simulink model "model_spis"  (R2016b)
settings: Solver=FixedStepDiscrete  StartTime=0.0  StopTime=inf  FixedStep=sampleTime  RelTol=1e-3
PostLoadFcn:
  | parameters_spis;
  | 
  | % set requested state
  | set_param('model_spis/Requested state','Value',num2str(0));
InitFcn:
  | parameters_spis;
  | 
  | % set requested state
  | set_param('model_spis/Requested state','Value',num2str(0));
StartFcn:
  | parameters_spis;
  | 
  | % set requested state
  | set_param('model_spis/Requested state','Value',num2str(0));
undefined symbols (not defined in the file): FM1, FM2, Lb, Lf, Lu, sampleTime
libraries: simulink x29, LibraryFM x14, VariousBlocksLibrary x7, simulink_extras x1
(part 1 of 3)
settings Model: SimulationMode=external  Creator=niekbeckers  LastModifiedBy=Labuser
settings DataIOCC: LimitDataPoints=on  SaveFormat=Array
settings OptimizationCC: BlockReduction=off  BooleanDataType=off  LocalBlockOutputs=off  LifeSpan=inf
settings DebuggingCC: SaveWithParameterizedLinksMsg=none  UnderspecifiedInitializationDetection=Classic  MergeDetectMultiDrivingBlocksExec=none  SignalResolutionControl=TryResolveAllWithWarning  SFUnexpectedBacktrackingDiag=warning  SFNoUnconditionalDefaultTransitionDiag=warning  SFExecutionAtInitializationDiag=none
settings HardwareCC: ProdBitPerPointer=32  ProdBitPerSizeT=32  ProdBitPerPtrDiffT=32  ProdLargestAtomicFloat=None  ProdIntDivRoundTo=Undefined  ProdEndianess=Unspecified  ProdWordSize=32  ProdHWDeviceType=32-bit Generic  TargetBitPerPointer=64  TargetBitPerSizeT=64  TargetBitPerPtrDiffT=64  TargetLongLongMode=on  TargetIntDivRoundTo=Zero  TargetEndianess=LittleEndian  TargetWordSize=64  TargetHWDeviceType=MATLAB Host  ProdEqTarget=off
settings ModelReferenceCC: PropagateSignalLabelsOutOfModel=off
settings RTWCC: SystemTargetFile=TwinCAT.tlc  GenCodeOnly=on  MakeCommand=make_tct  TemplateMakefile=tct_msbuild.tmf  Description=TwinCAT Target  GenerateReport=on  TargetLang=C++
settings STFCustomTargetCC: CompOptLevelCompliant=on  GeneratePreprocessorConditionals=Disable all  MATLABClassNameForMDSCustomization=Simulink.SoftwareTarget.TargetSpecificTriggerConfigurationBase  SystemTargetFile=TwinCAT.tlc
settings ConfigComp: CovMetricSettings=dw  CovHtmlReporting=on  CovSaveCumulativeToWorkspaceVar=on  CovSaveSingleToWorkspaceVar=on  CovExternalEMLEnable=off  CovSFcnEnable=off

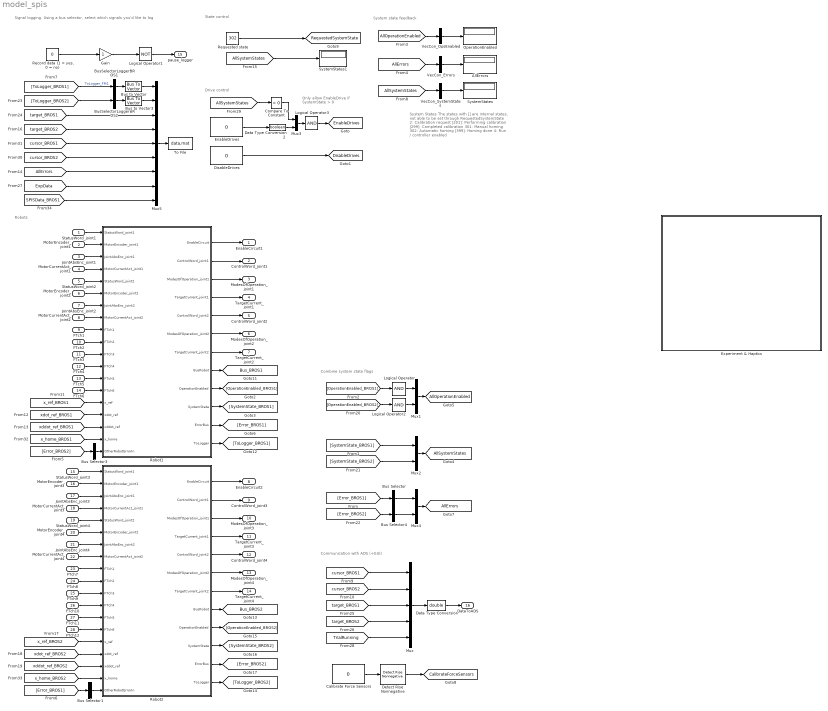
== system model_spis ==
  note: Drive control
  note: System state feedback
  note: Only allow EnableDrive
      | if SystemState > 0
  note: Communication with ADS (+GUI)
  note: Signal logging.
      | Using a bus selector, select which signals you'd like to log
  note: System States
      | The states with [] are internal states, not able to be set through RequestedSystemState
      | 2: Calibration request
      | [201]: Performing calibration
      | [299]: Completed calibration
      | 301: Manual homing
      | 302: Automatic homing
      | [399]: Homing done
      | 4: Run / controller enabled
  note: State control
  note: Combine system state flags
  note: Robots
  StatusWord_joint1 : Inport  OutDataTypeStr=uint16  PortDimensions=1
  MotorEncoder_joint1 : Inport  Port=2  OutDataTypeStr=int32  PortDimensions=1
  JointAbsEnc_joint1 : Inport  Port=3  OutDataTypeStr=int32  PortDimensions=1
  MotorCurrentAct_joint1 : Inport  Port=4  OutDataTypeStr=int16  PortDimensions=1
  StatusWord_joint2 : Inport  Port=5  OutDataTypeStr=uint16  PortDimensions=1
  MotorEncoder_joint2 : Inport  Port=6  OutDataTypeStr=int32  PortDimensions=1
  JointAbsEnc_joint2 : Inport  Port=7  OutDataTypeStr=int32  PortDimensions=1
  MotorCurrentAct_joint2 : Inport  Port=8  OutDataTypeStr=int16  PortDimensions=1
  FTch1 : Inport  Port=9  OutDataTypeStr=single  PortDimensions=1
  FTch2 : Inport  Port=10  OutDataTypeStr=single  PortDimensions=1
  FTch3 : Inport  Port=11  OutDataTypeStr=single  PortDimensions=1
  FTch4 : Inport  Port=12  OutDataTypeStr=single  PortDimensions=1
  FTch5 : Inport  Port=13  OutDataTypeStr=single  PortDimensions=1
  FTch6 : Inport  Port=14  OutDataTypeStr=single  PortDimensions=1
  StatusWord_joint3 : Inport  Port=15  OutDataTypeStr=uint16  PortDimensions=1
  MotorEncoder_joint3 : Inport  Port=16  OutDataTypeStr=int32  PortDimensions=1
  JointAbsEnc_joint3 : Inport  Port=17  OutDataTypeStr=int32  PortDimensions=1
  MotorCurrentAct_joint3 : Inport  Port=18  OutDataTypeStr=int16  PortDimensions=1
  StatusWord_joint4 : Inport  Port=19  OutDataTypeStr=uint16  PortDimensions=1
  MotorEncoder_joint4 : Inport  Port=20  OutDataTypeStr=int32  PortDimensions=1
  JointAbsEnc_joint4 : Inport  Port=21  OutDataTypeStr=int32  PortDimensions=1
  MotorCurrentAct_joint4 : Inport  Port=22  OutDataTypeStr=int16  PortDimensions=1
  FTch7 : Inport  Port=23  OutDataTypeStr=single  PortDimensions=1
  FTch8 : Inport  Port=24  OutDataTypeStr=single  PortDimensions=1
  FTch9 : Inport  Port=25  OutDataTypeStr=single  PortDimensions=1
  FTch10 : Inport  Port=26  OutDataTypeStr=single  PortDimensions=1
  FTch11 : Inport  Port=27  OutDataTypeStr=single  PortDimensions=1
  FTch12 : Inport  Port=28  OutDataTypeStr=single  PortDimensions=1
  AllErrors : Display
  Bus Selector : BusSelector  OutputSignals=ErrorCodeLatched  OutputAsBus=on
  Bus Selector1 : BusSelector  OutputSignals=ErrorCode  OutputAsBus=on
  Bus Selector3 : BusSelector  OutputSignals=ErrorCode  OutputAsBus=on
  Bus Selector4 : BusSelector  OutputSignals=ErrorCodeLatched  OutputAsBus=on
  Bus to Vector : BusToVector
  Bus to Vector3 : BusToVector
  BusSelectorLoggerBROS1 : BusSelector  OutputSignals=SystemState,qJointSpace.q_AbsEnc,qJointSpace.qdot_AbsEnc,qJointSpace.q_IncEnc,qJointSpace.qdot_IncEnc,xOpSpace.x_AbsEnc,xOpSpace.xdot_AbsEnc,Controller_ToLogger.x_ref,Controller_ToLogger.xdot_ref,Controller_ToLogger.xddot_ref,qJointSpace.JointTorque_Nm,BusFTSensor.ForcesOpSpace,BusActuators.BusActuator1.JointVelocity_LPF_rads,BusActuators.BusActuator2.JointVelocity_LPF_rads  OutputAsBus=on
  BusSelectorLoggerBROS2 : BusSelector  OutputSignals=SystemState,qJointSpace.q_AbsEnc,qJointSpace.qdot_AbsEnc,qJointSpace.q_IncEnc,qJointSpace.qdot_IncEnc,xOpSpace.x_AbsEnc,xOpSpace.xdot_AbsEnc,Controller_ToLogger.x_ref,Controller_ToLogger.xdot_ref,Controller_ToLogger.xddot_ref,qJointSpace.JointTorque_Nm,BusFTSensor.ForcesOpSpace,BusActuators.BusActuator1.JointVelocity_LPF_rads,BusActuators.BusActuator2.JointVelocity_LPF_rads  OutputAsBus=on
  Calibrate Force Sensors : Constant  Value=0
      settings: OpenFcn=set_param(gcb,'Value','1');tname = ['toggletimer_' gcb];delete(timerfind('name',tname));t = timer('timerfcn', ['set_param(''',gcb,''',''Value'',''0'')'],'executionmode','singleshot','startdelay',1,'name',tname);start(t);
      mask Display: fprintf('PushToTrigger\n%s',get_param(gcb,'value'))
  Compare To Constant : simulink/Logic and Bit Operations/Compare To Constant  relop=>  const=0  OutDataTypeStr=boolean
  Data Type Conversion : DataTypeConversion  OutDataTypeStr=double
  Data Type Conversion2 : DataTypeConversion  OutDataTypeStr=boolean
  Detect Rise Nonnegative : simulink/Logic and Bit Operations/Detect Rise Nonnegative  vinit=0  OutDataTypeStr=boolean
  DisableDrives : Constant  Value=0
      settings: OpenFcn=set_param(gcb,'Value','1');tname = ['toggletimer_' gcb];delete(timerfind('name',tname));t = timer('timerfcn', ['set_param(''',gcb,''',''Value'',''0'')'],'executionmode','singleshot','startdelay',1,'name',tname);start(t);
      mask Display: fprintf('PushToTrigger\n%s',get_param(gcb,'value'))
  EnableDrives : Constant  Value=0
      settings: OpenFcn=set_param(gcb,'Value','1');tname = ['toggletimer_' gcb];delete(timerfind('name',tname));t = timer('timerfcn', ['set_param(''',gcb,''',''Value'',''0'')'],'executionmode','singleshot','startdelay',1,'name',tname);start(t);
      mask Display: fprintf('PushToTrigger\n%s',get_param(gcb,'value'))
  Experiment & Haptics : Subsystem
  Gain : Gain
  Logical Operator : Logic  Inputs=1  AllPortsSameDT=off  OutDataTypeStr=boolean
  Logical Operator1 : Logic  Operator=NOT  Inputs=1  AllPortsSameDT=off  OutDataTypeStr=boolean
  Logical Operator2 : Logic  Inputs=1  AllPortsSameDT=off  OutDataTypeStr=boolean
  Logical Operator3 : Logic  Inputs=1  AllPortsSameDT=off  OutDataTypeStr=boolean
  Mux : Mux  Inputs=5
  Mux{1..4} (4 alike) : Mux  Inputs=2
  Mux5 : Mux  Inputs=9
  OperationEnabled : Display
  "Record data (1 = yes, 0 = no)" : Constant  Value=0
  Requested state : Constant  Value=302
  Robot1 : Subsystem  mask{RobotStruct=FM1}
      mask prompts: RobotStruct "Robot struct (data)"
  Robot2 : Subsystem  mask{RobotStruct=FM2}
      mask prompts: RobotStruct "Robot struct (data)"
  SystemStates : Display
  SystemStates1 : Display
  To File : ToFile  Filename=data.mat  MatrixName=data
  VecCon_Errors : Concatenate  NumInputs=1
  VecCon_OpsEnabled : Concatenate  NumInputs=1
  VecCon_SystemStates : Concatenate  NumInputs=1
  EnableCircuit1 : Outport  OutDataTypeStr=boolean  PortDimensions=1
  ControlWord_joint1 : Outport  Port=2  OutDataTypeStr=uint16  PortDimensions=1
  ModesOfOperation_joint1 : Outport  Port=3  OutDataTypeStr=int8  PortDimensions=1
  TargetCurrent_joint1 : Outport  Port=4  OutDataTypeStr=int16  PortDimensions=1
  ControlWord_joint2 : Outport  Port=5  OutDataTypeStr=uint16  PortDimensions=1
  ModesOfOperation_joint2 : Outport  Port=6  OutDataTypeStr=int8  PortDimensions=1
  TargetCurrent_joint2 : Outport  Port=7  OutDataTypeStr=int16  PortDimensions=1
  EnableCircuit2 : Outport  Port=8  OutDataTypeStr=boolean  PortDimensions=1
  ControlWord_joint3 : Outport  Port=9  OutDataTypeStr=uint16  PortDimensions=1
  ModesOfOperation_joint3 : Outport  Port=10  OutDataTypeStr=int8  PortDimensions=1
  TargetCurrent_joint3 : Outport  Port=11  OutDataTypeStr=int16  PortDimensions=1
  ControlWord_joint4 : Outport  Port=12  OutDataTypeStr=uint16  PortDimensions=1
  ModesOfOperation_joint4 : Outport  Port=13  OutDataTypeStr=int8  PortDimensions=1
  TargetCurrent_joint4 : Outport  Port=14  OutDataTypeStr=int16  PortDimensions=1
  pause_logger : Outport  Port=15  OutDataTypeStr=boolean  PortDimensions=1
  DataToADS : Outport  Port=16  OutDataTypeStr=double
  tag scope: AllErrors=global, AllOperationEnabled=global, AllSystemStates=global, Bus_BROS1=global, Bus_BROS2=global, CalibrateForceSensors=global, DisableDrives=global, EnableDrives=global, RequestedSystemState=global
  wires:
  DisableDrives/1 -> [DisableDrives]
  Robot1/9(OperationEnabled) -> [OperationEnabled_BROS1]
  [AllOperationEnabled] -> VecCon_OpsEnabled/1
  Robot1/10(SystemState) -> [SystemState_BROS1]
  [SystemState_BROS1] -> Mux2/1
  Mux2/1 -> [AllSystemStates]
  Mux1/1 -> [AllOperationEnabled]
  [OperationEnabled_BROS1] -> Logical Operator/1
  Robot1/11(ErrorBus) -> [Error_BROS1]
  [Error_BROS1] -> Bus Selector/1
  [AllErrors] -> VecCon_Errors/1
  [x_ref_BROS1] -> Robot1/15(x_ref)
  [xdot_ref_BROS1] -> Robot1/16(xdot_ref)
  [xddot_ref_BROS1] -> Robot1/17(xddot_ref)
  Requested state/1 -> [RequestedSystemState]
  Robot1/8(BusRobot) -> [Bus_BROS1]
  StatusWord_joint1/1 -> Robot1/1(StatusWord_joint1)
  MotorEncoder_joint1/1 -> Robot1/2(MotorEncoder_joint1)
  JointAbsEnc_joint1/1 -> Robot1/3(JointAbsEnc_joint1)
  MotorCurrentAct_joint1/1 -> Robot1/4(MotorCurrentAct_joint1)
  StatusWord_joint2/1 -> Robot1/5(StatusWord_joint2)
  MotorEncoder_joint2/1 -> Robot1/6(MotorEncoder_joint2)
  JointAbsEnc_joint2/1 -> Robot1/7(JointAbsEnc_joint2)
  MotorCurrentAct_joint2/1 -> Robot1/8(MotorCurrentAct_joint2)
  FTch1/1 -> Robot1/9(FTch1)
  FTch2/1 -> Robot1/10(FTch2)
  FTch3/1 -> Robot1/11(FTch3)
  FTch4/1 -> Robot1/12(FTch4)
  FTch5/1 -> Robot1/13(FTch5)
  FTch6/1 -> Robot1/14(FTch6)
  Robot1/2(ControlWord_joint1) -> ControlWord_joint1/1
  Robot1/3(ModesOfOperation_joint1) -> ModesOfOperation_joint1/1
  Robot1/4(TargetCurrent_joint1) -> TargetCurrent_joint1/1
  Robot1/7(TargetCurrent_joint2) -> TargetCurrent_joint2/1
  Robot1/6(ModesOfOperation_joint2) -> ModesOfOperation_joint2/1
  Robot1/5(ControlWord_joint2) -> ControlWord_joint2/1
  Robot1/12(ToLogger) -> [ToLogger_BROS1]
  [ToLogger_BROS1] -> BusSelectorLoggerBROS1/1  "ToLogger_FM1"
  Logical Operator/1 -> Mux1/1
  [AllSystemStates] -> SystemStates1/1
  Logical Operator1/1 -> pause_logger/1
  BusSelectorLoggerBROS1/1 -> Bus to Vector/1
  Robot2/9(OperationEnabled) -> [OperationEnabled_BROS2]
  Robot2/10(SystemState) -> [SystemState_BROS2]
  Robot2/11(ErrorBus) -> [Error_BROS2]
  [x_ref_BROS2] -> Robot2/15(x_ref)
  [xdot_ref_BROS2] -> Robot2/16(xdot_ref)
  [xddot_ref_BROS2] -> Robot2/17(xddot_ref)
  Robot2/8(BusRobot) -> [Bus_BROS2]
  StatusWord_joint3/1 -> Robot2/1(StatusWord_joint1)
  MotorEncoder_joint3/1 -> Robot2/2(MotorEncoder_joint1)
  JointAbsEnc_joint3/1 -> Robot2/3(JointAbsEnc_joint1)
  MotorCurrentAct_joint3/1 -> Robot2/4(MotorCurrentAct_joint1)
  StatusWord_joint4/1 -> Robot2/5(StatusWord_joint2)
  MotorEncoder_joint4/1 -> Robot2/6(MotorEncoder_joint2)
  MotorCurrentAct_joint4/1 -> Robot2/8(MotorCurrentAct_joint2)
  FTch7/1 -> Robot2/9(FTch1)
  FTch8/1 -> Robot2/10(FTch2)
  FTch9/1 -> Robot2/11(FTch3)
  FTch10/1 -> Robot2/12(FTch4)
  FTch12/1 -> Robot2/14(FTch6)
  Robot2/1(EnableCircuit) -> EnableCircuit2/1
  Robot2/2(ControlWord_joint1) -> ControlWord_joint3/1
  Robot2/3(ModesOfOperation_joint1) -> ModesOfOperation_joint3/1
  Robot2/7(TargetCurrent_joint2) -> TargetCurrent_joint4/1
  Robot2/6(ModesOfOperation_joint2) -> ModesOfOperation_joint4/1
  Robot2/5(ControlWord_joint2) -> ControlWord_joint4/1
  Robot2/12(ToLogger) -> [ToLogger_BROS2]
  [OperationEnabled_BROS2] -> Logical Operator2/1
  Logical Operator2/1 -> Mux1/2
  [SystemState_BROS2] -> Mux2/2
  Mux4/1 -> [AllErrors]
  Bus Selector/1 -> Mux4/1
  [Error_BROS2] -> Bus Selector4/1
  Bus Selector4/1 -> Mux4/2
  [ToLogger_BROS2] -> BusSelectorLoggerBROS2/1
  BusSelectorLoggerBROS2/1 -> Bus to Vector3/1
  Bus to Vector3/1 -> Mux5/2
  Bus to Vector/1 -> Mux5/1
  Mux5/1 -> To File/1
  Robot1/1(EnableCircuit) -> EnableCircuit1/1
  Robot2/4(TargetCurrent_joint1) -> TargetCurrent_joint3/1
  JointAbsEnc_joint4/1 -> Robot2/7(JointAbsEnc_joint2)
  FTch11/1 -> Robot2/13(FTch5)
  [Error_BROS2] -> Bus Selector3/1
  [Error_BROS1] -> Bus Selector1/1
  Bus Selector1/1 -> Robot2/19(OtherRobotErrorIn)
  Bus Selector3/1 -> Robot1/19(OtherRobotErrorIn)
  VecCon_Errors/1 -> AllErrors/1
  [AllSystemStates] -> VecCon_SystemStates/1
  VecCon_SystemStates/1 -> SystemStates/1
  VecCon_OpsEnabled/1 -> OperationEnabled/1
  Mux/1 -> Data Type Conversion/1
  Data Type Conversion/1 -> DataToADS/1
  [cursor_BROS1] -> Mux/1
  [cursor_BROS2] -> Mux/2
  [target_BROS1] -> Mux/3
  [target_BROS2] -> Mux/4
  [TrialRunning] -> Mux/5
  Calibrate Force Sensors/1 -> Detect Rise Nonnegative/1
  Detect Rise Nonnegative/1 -> [CalibrateForceSensors]
  [target_BROS1] -> Mux5/3
  [AllErrors] -> Mux5/7
  [ExpData] -> Mux5/8
  [target_BROS2] -> Mux5/4
  [AllSystemStates] -> Compare To Constant/1
  Logical Operator3/1 -> [EnableDrives]
  EnableDrives/1 -> Data Type Conversion2/1
  Compare To Constant/1 -> Mux3/1
  Mux3/1 -> Logical Operator3/1
  Data Type Conversion2/1 -> Mux3/2
  [cursor_BROS2] -> Mux5/6
  [cursor_BROS1] -> Mux5/5
  [x_home_BROS1] -> Robot1/18(x_home)
  [x_home_BROS2] -> Robot2/18(x_home)
  "Record data (1 = yes, 0 = no)"/1 -> Gain/1
  Gain/1 -> Logical Operator1/1
  [SPISData_BROS1] -> Mux5/9

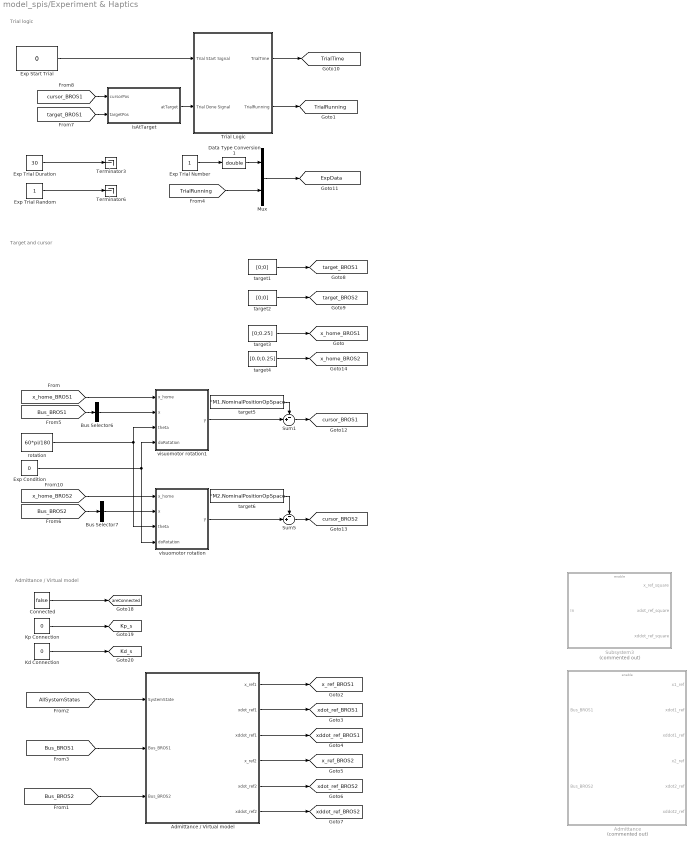
== system model_spis/Experiment & Haptics ==
  note: Target and cursor
  note: Trial logic
  note: Admittance / Virtual model
  Admittance : Subsystem  Commented=on
  Admittance / Virtual model : Subsystem
  Bus Selector6 : BusSelector  OutputSignals=xOpSpace.x  OutputAsBus=on
  Bus Selector7 : BusSelector  OutputSignals=xOpSpace.x  OutputAsBus=on
  Connected : Constant  Value=false  OutDataTypeStr=boolean
  Data Type Conversion1 : DataTypeConversion  OutDataTypeStr=double
  Exp Condition : Constant  Value=0  OutDataTypeStr=int32
  Exp Start Trial : Constant  Value=0
      settings: OpenFcn=set_param(gcb,'Value','1');tname = ['toggletimer_' gcb];delete(timerfind('name',tname));t = timer('timerfcn', ['set_param(''',gcb,''',''Value'',''0'')'],'executionmode','singleshot','startdelay',1,'name',tname);start(t);
      mask Display: fprintf('PushToTrigger\n%s',get_param(gcb,'value'))
  Exp Trial Duration : Constant  Value=30  OutDataTypeStr=double
  Exp Trial Number : Constant  OutDataTypeStr=int32
  Exp Trial Random : Constant  OutDataTypeStr=int32
  Kd Connection : Constant  Value=0  OutDataTypeStr=double
  Kp Connection : Constant  Value=0  OutDataTypeStr=double
  Mux : Mux  Inputs=2
  Subsystem3 : Subsystem  Commented=on
  Sum1 : Sum  Inputs=-+|
  Sum5 : Sum  Inputs=-+|
  Terminator3 : Terminator
  Terminator6 : Terminator
  Trial Logic : Subsystem
  isAtTarget : MATLAB Function  TreatAsAtomicUnit=on
  rotation : Constant  Value=60*pi/180  OutDataTypeStr=double
  target1 : Constant  Value=[0;0]
  target2 : Constant  Value=[0;0]
  target3 : Constant  Value=[0;0.25]
  target4 : Constant  Value=[0.0;0.25]
  target5 : Constant  Value=FM1.NominalPositionOpSpace
  target6 : Constant  Value=FM2.NominalPositionOpSpace
  visuomotor rotation : MATLAB Function  TreatAsAtomicUnit=on
  visuomotor rotation1 : MATLAB Function  TreatAsAtomicUnit=on
  tag scope: ExpData=global, Kd_s=global, Kp_s=global, TrialRunning=global, TrialTime=global, areConnected=global, cursor_BROS1=global, cursor_BROS2=global, target_BROS1=global, target_BROS2=global, x_home_BROS1=global, x_home_BROS2=global, x_ref_BROS1=global, x_ref_BROS2=global, xddot_ref_BROS1=global, xddot_ref_BROS2=global, xdot_ref_BROS1=global, xdot_ref_BROS2=global
  wires:
  target2/1 -> [target_BROS2]
  Kp Connection/1 -> [Kp_s]
  Mux/1 -> [ExpData]
  Exp Trial Number/1 -> Data Type Conversion1/1
  [TrialRunning] -> Mux/2
  Connected/1 -> [areConnected]
  Exp Trial Random/1 -> Terminator6/1
  Data Type Conversion1/1 -> Mux/1
  Kd Connection/1 -> [Kd_s]
  [Bus_BROS1] -> Admittance / Virtual model/2(Bus_BROS1)
  [AllSystemStates] -> Admittance / Virtual model/1(SystemState)
  [Bus_BROS1] -> Bus Selector6/1
  [Bus_BROS2] -> Bus Selector7/1
  Exp Condition/1 -> visuomotor rotation1/4(doRotation), visuomotor rotation/4(doRotation)
  rotation/1 -> visuomotor rotation1/3(theta), visuomotor rotation/3(theta)
  Exp Trial Duration/1 -> Terminator3/1
  Bus Selector6/1 -> visuomotor rotation1/2(x)
  Bus Selector7/1 -> visuomotor rotation/2(x)
  [x_home_BROS1] -> visuomotor rotation1/1(x_home)
  target1/1 -> [target_BROS1]
  target3/1 -> [x_home_BROS1]
  target4/1 -> [x_home_BROS2]
  Exp Start Trial/1 -> Trial Logic/1(Trial Start Signal)
  Trial Logic/1(TrialTime) -> [TrialTime]
  Trial Logic/2(TrialRunning) -> [TrialRunning]
  [cursor_BROS1] -> isAtTarget/1(cursorPos)
  [target_BROS1] -> isAtTarget/2(targetPos)
  isAtTarget/1(atTarget) -> Trial Logic/2(Trial Done Signal)
  [Bus_BROS2] -> Admittance / Virtual model/3(Bus_BROS2)
  Admittance / Virtual model/1(x_ref1) -> [x_ref_BROS1]
  Admittance / Virtual model/2(xdot_ref1) -> [xdot_ref_BROS1]
  Admittance / Virtual model/3(xddot_ref1) -> [xddot_ref_BROS1]
  Admittance / Virtual model/4(x_ref2) -> [x_ref_BROS2]
  Admittance / Virtual model/5(xdot_ref2) -> [xdot_ref_BROS2]
  Admittance / Virtual model/6(xddot_ref2) -> [xddot_ref_BROS2]
  Sum1/1 -> [cursor_BROS1]
  visuomotor rotation/1(y) -> Sum5/2
  target6/1 -> Sum5/1
  Sum5/1 -> [cursor_BROS2]
  [x_home_BROS2] -> visuomotor rotation/1(x_home)
  visuomotor rotation1/1(y) -> Sum1/2
  target5/1 -> Sum1/1

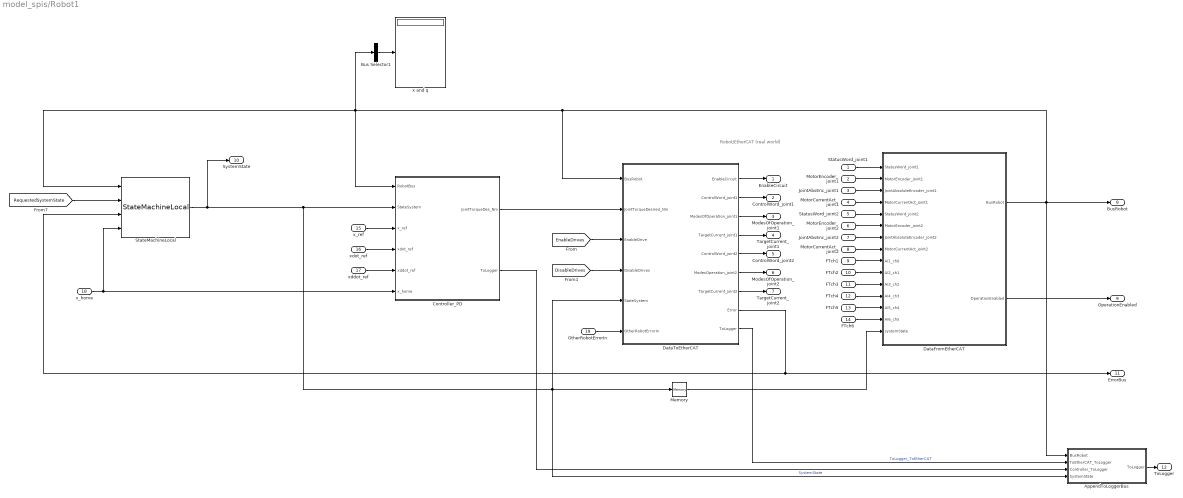
== system model_spis/Robot1 ==
  note: Robot/EtherCAT (real world)
  StatusWord_joint1 : Inport
  MotorEncoder_joint1 : Inport  Port=2
  JointAbsEnc_joint1 : Inport  Port=3
  MotorCurrentAct_joint1 : Inport  Port=4
  StatusWord_joint2 : Inport  Port=5
  MotorEncoder_joint2 : Inport  Port=6
  JointAbsEnc_joint2 : Inport  Port=7
  MotorCurrentAct_joint2 : Inport  Port=8
  FTch1 : Inport  Port=9
  FTch2 : Inport  Port=10
  FTch3 : Inport  Port=11
  FTch4 : Inport  Port=12
  FTch5 : Inport  Port=13
  FTch6 : Inport  Port=14
  x_ref : Inport  Port=15
  xdot_ref : Inport  Port=16
  xddot_ref : Inport  Port=17
  x_home : Inport  Port=18
  OtherRobotErrorIn : Inport  Port=19
  AppendToLoggerBus : Subsystem
  Bus Selector1 : BusSelector  OutputSignals=qJointSpace.q_AbsEnc,qJointSpace.qdot_AbsEnc,xOpSpace.x,BusActuators.BusActuator1.JointPosition_AbsEnc_rad,BusActuators.BusActuator2.JointPosition_AbsEnc_rad  OutputAsBus=on
  Controller_PD : Subsystem
  DataFromEtherCAT : Subsystem
  DataToEtherCAT : Subsystem
  Memory : Memory
  StateMachineLocal : LibraryFM/StateMachineLocal
  x and q : Display
  EnableCircuit : Outport
  ControlWord_joint1 : Outport  Port=2
  ModesOfOperation_joint1 : Outport  Port=3
  TargetCurrent_joint1 : Outport  Port=4
  ControlWord_joint2 : Outport  Port=5
  ModesOfOperation_joint2 : Outport  Port=6
  TargetCurrent_joint2 : Outport  Port=7
  BusRobot : Outport  Port=8
  OperationEnabled : Outport  Port=9
  SystemState : Outport  Port=10
  ErrorBus : Outport  Port=11
  ToLogger : Outport  Port=12
  wires:
  xddot_ref/1 -> Controller_PD/5(xddot_ref)
  xdot_ref/1 -> Controller_PD/4(xdot_ref)
  x_ref/1 -> Controller_PD/3(x_ref)
  DataToEtherCAT/7(TargetCurrent_joint2) -> TargetCurrent_joint2/1
  FTch2/1 -> DataFromEtherCAT/10(AI2_ch1)
  MotorCurrentAct_joint1/1 -> DataFromEtherCAT/4(MotorCurrentAct_joint1)
  MotorEncoder_joint2/1 -> DataFromEtherCAT/6(MotorEncoder_joint2)
  JointAbsEnc_joint1/1 -> DataFromEtherCAT/3(JointAbsoluteEncoder_joint1)
  DataToEtherCAT/3(ModesOfOperation_joint1) -> ModesOfOperation_joint1/1
  DataToEtherCAT/1(EnableCircuit) -> EnableCircuit/1
  FTch1/1 -> DataFromEtherCAT/9(AI1_ch0)
  StateMachineLocal/1 -> Controller_PD/2(StateSystem), DataToEtherCAT/5(StateSystem), Memory/1, AppendToLoggerBus/4(SystemState), SystemState/1  "SystemState"
  DataToEtherCAT/2(ControlWord_joint1) -> ControlWord_joint1/1
  DataToEtherCAT/8(Error) -> StateMachineLocal/3, ErrorBus/1
  DataFromEtherCAT/1(BusRobot) -> AppendToLoggerBus/1(BusRobot), Controller_PD/1(RobotBus), Bus Selector1/1, StateMachineLocal/1, DataToEtherCAT/1(BusRobot), BusRobot/1
  [RequestedSystemState] -> StateMachineLocal/2
  Controller_PD/1(JointTorqueDes_Nm) -> DataToEtherCAT/2(JointTorqueDesired_Nm)
  [DisableDrives] -> DataToEtherCAT/4(DisableDrives)
  [EnableDrives] -> DataToEtherCAT/3(EnableDrive)
  MotorCurrentAct_joint2/1 -> DataFromEtherCAT/8(MotorCurrentAct_joint2)
  DataToEtherCAT/4(TargetCurrent_joint1) -> TargetCurrent_joint1/1
  FTch5/1 -> DataFromEtherCAT/13(AI5_ch4)
  JointAbsEnc_joint2/1 -> DataFromEtherCAT/7("JointAbsoluteEncoder_joint2 ")
  MotorEncoder_joint1/1 -> DataFromEtherCAT/2(MotorEncoder_joint1)
  DataToEtherCAT/5(ControlWord_joint2) -> ControlWord_joint2/1
  DataToEtherCAT/6(ModesOperation_joint2) -> ModesOfOperation_joint2/1
  StatusWord_joint1/1 -> DataFromEtherCAT/1(StatusWord_joint1)
  StatusWord_joint2/1 -> DataFromEtherCAT/5(StatusWord_joint2)
  FTch6/1 -> DataFromEtherCAT/14(AI6_ch5)
  FTch4/1 -> DataFromEtherCAT/12(AI4_ch3)
  FTch3/1 -> DataFromEtherCAT/11(AI3_ch2)
  DataFromEtherCAT/2(OperationEnabled) -> OperationEnabled/1
  Bus Selector1/1 -> x and q/1
  Controller_PD/2(ToLogger) -> AppendToLoggerBus/3(Controller_ToLogger)
  DataToEtherCAT/9(ToLogger) -> AppendToLoggerBus/2(ToEtherCAT_ToLogger)  "ToLogger_ToEtherCAT"
  AppendToLoggerBus/1(ToLogger) -> ToLogger/1
  Memory/1 -> DataFromEtherCAT/15(systemState)
  OtherRobotErrorIn/1 -> DataToEtherCAT/6(OtherRobotErrorIn)
  x_home/1 -> StateMachineLocal/4, Controller_PD/6(x_home)

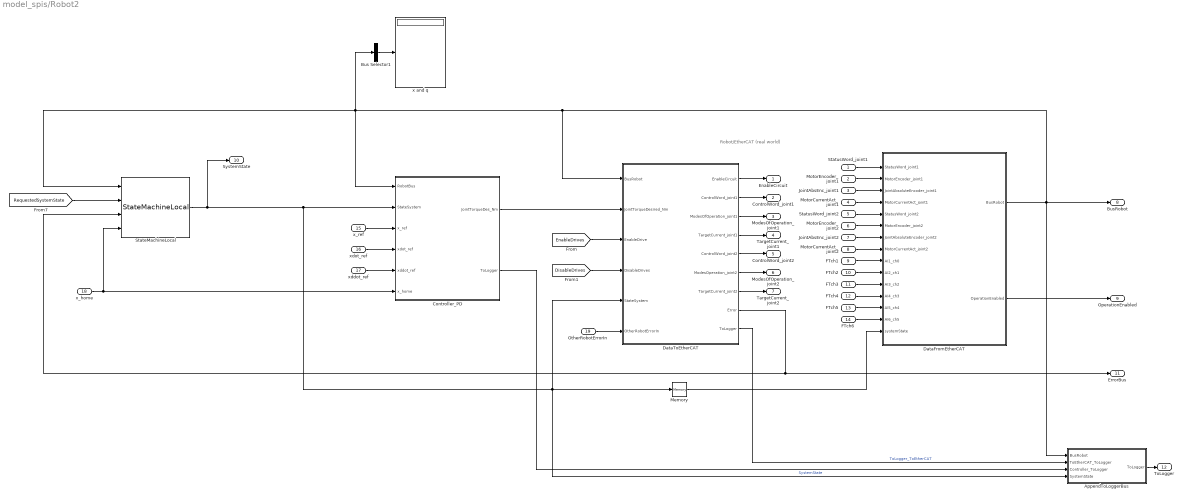
== system model_spis/Robot2 ==
  note: Robot/EtherCAT (real world)
  StatusWord_joint1 : Inport
  MotorEncoder_joint1 : Inport  Port=2
  JointAbsEnc_joint1 : Inport  Port=3
  MotorCurrentAct_joint1 : Inport  Port=4
  StatusWord_joint2 : Inport  Port=5
  MotorEncoder_joint2 : Inport  Port=6
  JointAbsEnc_joint2 : Inport  Port=7
  MotorCurrentAct_joint2 : Inport  Port=8
  FTch1 : Inport  Port=9
  FTch2 : Inport  Port=10
  FTch3 : Inport  Port=11
  FTch4 : Inport  Port=12
  FTch5 : Inport  Port=13
  FTch6 : Inport  Port=14
  x_ref : Inport  Port=15
  xdot_ref : Inport  Port=16
  xddot_ref : Inport  Port=17
  x_home : Inport  Port=18
  OtherRobotErrorIn : Inport  Port=19
  AppendToLoggerBus : Subsystem
  Bus Selector1 : BusSelector  OutputSignals=qJointSpace.q_AbsEnc,qJointSpace.qdot_AbsEnc,xOpSpace.x,BusActuators.BusActuator1.JointPosition_AbsEnc_rad,BusActuators.BusActuator2.JointPosition_AbsEnc_rad  OutputAsBus=on
  Controller_PD : Subsystem
  DataFromEtherCAT : Subsystem
  DataToEtherCAT : Subsystem
  Memory : Memory
  StateMachineLocal : LibraryFM/StateMachineLocal
  x and q : Display
  EnableCircuit : Outport
  ControlWord_joint1 : Outport  Port=2
  ModesOfOperation_joint1 : Outport  Port=3
  TargetCurrent_joint1 : Outport  Port=4
  ControlWord_joint2 : Outport  Port=5
  ModesOfOperation_joint2 : Outport  Port=6
  TargetCurrent_joint2 : Outport  Port=7
  BusRobot : Outport  Port=8
  OperationEnabled : Outport  Port=9
  SystemState : Outport  Port=10
  ErrorBus : Outport  Port=11
  ToLogger : Outport  Port=12
  wires:
  xddot_ref/1 -> Controller_PD/5(xddot_ref)
  xdot_ref/1 -> Controller_PD/4(xdot_ref)
  x_ref/1 -> Controller_PD/3(x_ref)
  DataToEtherCAT/7(TargetCurrent_joint2) -> TargetCurrent_joint2/1
  FTch2/1 -> DataFromEtherCAT/10(AI2_ch1)
  MotorCurrentAct_joint1/1 -> DataFromEtherCAT/4(MotorCurrentAct_joint1)
  MotorEncoder_joint2/1 -> DataFromEtherCAT/6(MotorEncoder_joint2)
  JointAbsEnc_joint1/1 -> DataFromEtherCAT/3(JointAbsoluteEncoder_joint1)
  DataToEtherCAT/3(ModesOfOperation_joint1) -> ModesOfOperation_joint1/1
  DataToEtherCAT/1(EnableCircuit) -> EnableCircuit/1
  FTch1/1 -> DataFromEtherCAT/9(AI1_ch0)
  StateMachineLocal/1 -> Controller_PD/2(StateSystem), DataToEtherCAT/5(StateSystem), Memory/1, AppendToLoggerBus/4(SystemState), SystemState/1  "SystemState"
  DataToEtherCAT/2(ControlWord_joint1) -> ControlWord_joint1/1
  DataToEtherCAT/8(Error) -> StateMachineLocal/3, ErrorBus/1
  DataFromEtherCAT/1(BusRobot) -> AppendToLoggerBus/1(BusRobot), Controller_PD/1(RobotBus), Bus Selector1/1, StateMachineLocal/1, DataToEtherCAT/1(BusRobot), BusRobot/1
  [RequestedSystemState] -> StateMachineLocal/2
  Controller_PD/1(JointTorqueDes_Nm) -> DataToEtherCAT/2(JointTorqueDesired_Nm)
  [DisableDrives] -> DataToEtherCAT/4(DisableDrives)
  [EnableDrives] -> DataToEtherCAT/3(EnableDrive)
  MotorCurrentAct_joint2/1 -> DataFromEtherCAT/8(MotorCurrentAct_joint2)
  DataToEtherCAT/4(TargetCurrent_joint1) -> TargetCurrent_joint1/1
  FTch5/1 -> DataFromEtherCAT/13(AI5_ch4)
  JointAbsEnc_joint2/1 -> DataFromEtherCAT/7("JointAbsoluteEncoder_joint2 ")
  MotorEncoder_joint1/1 -> DataFromEtherCAT/2(MotorEncoder_joint1)
  DataToEtherCAT/5(ControlWord_joint2) -> ControlWord_joint2/1
  DataToEtherCAT/6(ModesOperation_joint2) -> ModesOfOperation_joint2/1
  StatusWord_joint1/1 -> DataFromEtherCAT/1(StatusWord_joint1)
  StatusWord_joint2/1 -> DataFromEtherCAT/5(StatusWord_joint2)
  FTch6/1 -> DataFromEtherCAT/14(AI6_ch5)
  FTch4/1 -> DataFromEtherCAT/12(AI4_ch3)
  FTch3/1 -> DataFromEtherCAT/11(AI3_ch2)
  DataFromEtherCAT/2(OperationEnabled) -> OperationEnabled/1
  Bus Selector1/1 -> x and q/1
  Controller_PD/2(ToLogger) -> AppendToLoggerBus/3(Controller_ToLogger)
  DataToEtherCAT/9(ToLogger) -> AppendToLoggerBus/2(ToEtherCAT_ToLogger)  "ToLogger_ToEtherCAT"
  AppendToLoggerBus/1(ToLogger) -> ToLogger/1
  Memory/1 -> DataFromEtherCAT/15(systemState)
  OtherRobotErrorIn/1 -> DataToEtherCAT/6(OtherRobotErrorIn)
  x_home/1 -> StateMachineLocal/4, Controller_PD/6(x_home)

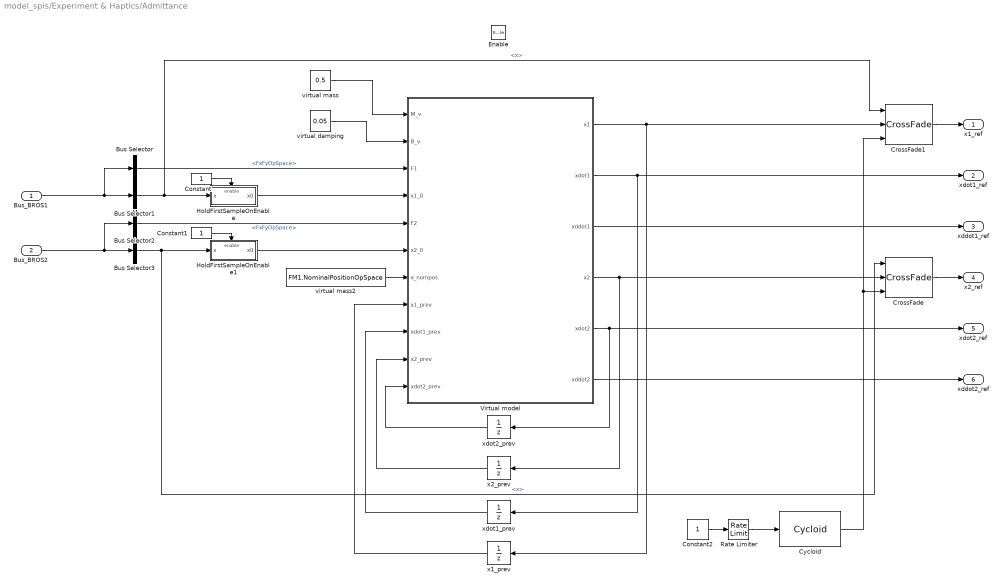
== system model_spis/Experiment & Haptics/Admittance ==
  Bus_BROS1 : Inport
  Bus_BROS2 : Inport  Port=2
  Enable : EnablePort  StatesWhenEnabling=reset
  Bus Selector : BusSelector  OutputSignals=BusFTSensor.FxFyOpSpace
  Bus Selector1 : BusSelector  OutputSignals=xOpSpace.x
  Bus Selector2 : BusSelector  OutputSignals=BusFTSensor.FxFyOpSpace
  Bus Selector3 : BusSelector  OutputSignals=xOpSpace.x
  Constant : Constant
  Constant1 : Constant
  Constant2 : Constant
  CrossFade : VariousBlocksLibrary/Various/CrossFade
  CrossFade1 : VariousBlocksLibrary/Various/CrossFade
  Cycloid : VariousBlocksLibrary/Various/Cycloid
  HoldFirstSampleOnEnable : Subsystem
  HoldFirstSampleOnEnable1 : Subsystem
  Rate Limiter : RateLimiter  FallingSlewLimit=-0.2  SampleTimeMode=inherited
  Virtual model : MATLAB Function  TreatAsAtomicUnit=on
  virtual damping : Constant  Value=0.05
  virtual mass : Constant  Value=0.5
  virtual mass2 : Constant  Value=FM1.NominalPositionOpSpace
  x1_prev : UnitDelay  SampleTime=-1
  x2_prev : UnitDelay  SampleTime=-1
  xdot1_prev : UnitDelay  SampleTime=-1
  xdot2_prev : UnitDelay  SampleTime=-1
  x1_ref : Outport
  xdot1_ref : Outport  Port=2
  xddot1_ref : Outport  Port=3
  x2_ref : Outport  Port=4
  xdot2_ref : Outport  Port=5
  xddot2_ref : Outport  Port=6
  wires:
  virtual mass2/1 -> Virtual model/7(x_nompos)
  HoldFirstSampleOnEnable/1(x0) -> Virtual model/4(x1_0)
  Bus Selector1/1 -> CrossFade1/1, HoldFirstSampleOnEnable/1(x)  "<x>"
  Constant/1 -> HoldFirstSampleOnEnable/Enable
  Bus Selector/1 -> Virtual model/3(F1)  "<FxFyOpSpace>"
  Bus_BROS1/1 -> Bus Selector/1, Bus Selector1/1
  virtual mass/1 -> Virtual model/1(M_v)
  Virtual model/2(xdot1) -> xdot1_ref/1, xdot1_prev/1
  xdot1_prev/1 -> Virtual model/9(xdot1_prev)
  x1_prev/1 -> Virtual model/8(x1_prev)
  Virtual model/3(xddot1) -> xddot1_ref/1
  Virtual model/1(x1) -> CrossFade1/2, x1_prev/1
  virtual damping/1 -> Virtual model/2(B_v)
  Virtual model/4(x2) -> CrossFade/2, x2_prev/1
  Virtual model/5(xdot2) -> xdot2_prev/1, xdot2_ref/1
  Virtual model/6(xddot2) -> xddot2_ref/1
  Bus Selector3/1 -> CrossFade/1, HoldFirstSampleOnEnable1/1(x)  "<x>"
  Constant1/1 -> HoldFirstSampleOnEnable1/Enable
  Bus Selector2/1 -> Virtual model/5(F2)  "<FxFyOpSpace>"
  Bus_BROS2/1 -> Bus Selector2/1, Bus Selector3/1
  HoldFirstSampleOnEnable1/1(x0) -> Virtual model/6(x2_0)
  x2_prev/1 -> Virtual model/10(x2_prev)
  xdot2_prev/1 -> Virtual model/11(xdot2_prev)
  Cycloid/1 -> CrossFade/3, CrossFade1/3
  Rate Limiter/1 -> Cycloid/1
  Constant2/1 -> Rate Limiter/1
  CrossFade/1 -> x2_ref/1
  CrossFade1/1 -> x1_ref/1

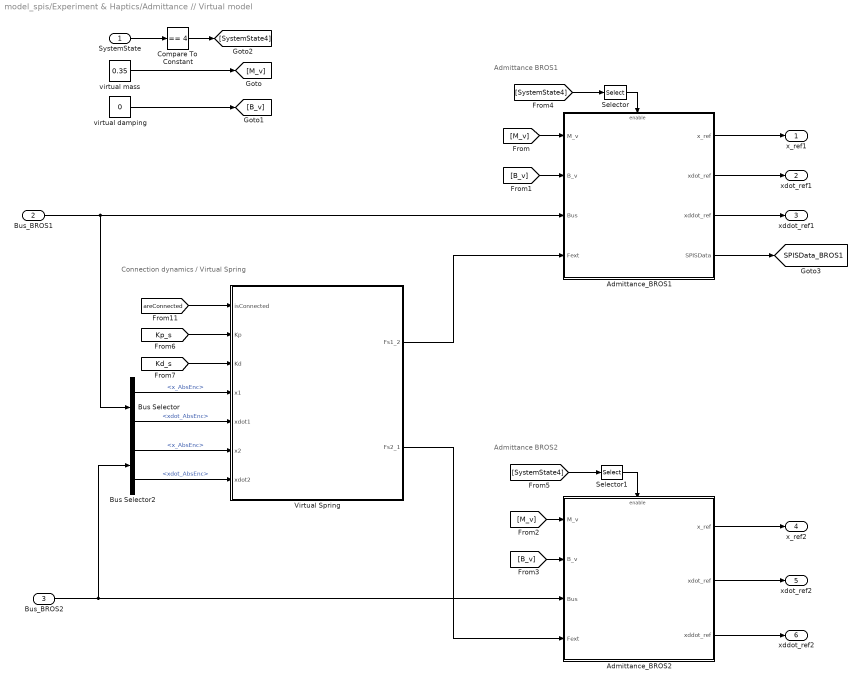
== system model_spis/Experiment & Haptics/Admittance // Virtual model ==
  note: Connection dynamics / Virtual Spring
  note: Admittance BROS2
  note: Admittance BROS1
  SystemState : Inport
  Bus_BROS1 : Inport  Port=2
  Bus_BROS2 : Inport  Port=3
  Admittance_BROS1 : Subsystem
  Admittance_BROS2 : Subsystem
  Bus Selector : BusSelector  OutputSignals=xOpSpace.x_AbsEnc,xOpSpace.xdot_AbsEnc
  Bus Selector2 : BusSelector  OutputSignals=xOpSpace.x_AbsEnc,xOpSpace.xdot_AbsEnc
  Compare To Constant : simulink/Logic and Bit Operations/Compare To Constant  relop===  const=4  OutDataTypeStr=boolean
  Selector : Selector  InputPortWidth=2  IndexOptions=Index vector (dialog)  Indices=1  OutputSizes=1
  Selector1 : Selector  InputPortWidth=2  IndexOptions=Index vector (dialog)  Indices=2  OutputSizes=1
  Virtual Spring : MATLAB Function  TreatAsAtomicUnit=on
  virtual damping : Constant  Value=0
  virtual mass : Constant  Value=0.35
  x_ref1 : Outport
  xdot_ref1 : Outport  Port=2
  xddot_ref1 : Outport  Port=3
  x_ref2 : Outport  Port=4
  xdot_ref2 : Outport  Port=5
  xddot_ref2 : Outport  Port=6
  tag scope: SPISData_BROS1=global
  wires:
  Bus_BROS2/1 -> Bus Selector2/1, Admittance_BROS2/3(Bus)
  Selector1/1 -> Admittance_BROS2/Enable
  Admittance_BROS2/1(x_ref) -> x_ref2/1
  Admittance_BROS1/1(x_ref) -> x_ref1/1
  Admittance_BROS2/2(xdot_ref) -> xdot_ref2/1
  Bus_BROS1/1 -> Bus Selector/1, Admittance_BROS1/3(Bus)
  Admittance_BROS1/2(xdot_ref) -> xdot_ref1/1
  Admittance_BROS1/3(xddot_ref) -> xddot_ref1/1
  Admittance_BROS2/3(xddot_ref) -> xddot_ref2/1
  SystemState/1 -> Compare To Constant/1
  Selector/1 -> Admittance_BROS1/Enable
  virtual mass/1 -> [M_v]
  virtual damping/1 -> [B_v]
  [M_v] -> Admittance_BROS1/1(M_v)
  [B_v] -> Admittance_BROS1/2(B_v)
  [M_v] -> Admittance_BROS2/1(M_v)
  [B_v] -> Admittance_BROS2/2(B_v)
  Compare To Constant/1 -> [SystemState4]
  [SystemState4] -> Selector/1
  [SystemState4] -> Selector1/1
  Virtual Spring/1(Fs1_2) -> Admittance_BROS1/4(Fext)
  Bus Selector/2 -> Virtual Spring/5(xdot1)  "<xdot_AbsEnc>"
  Bus Selector/1 -> Virtual Spring/4(x1)  "<x_AbsEnc>"
  Bus Selector2/1 -> Virtual Spring/6(x2)  "<x_AbsEnc>"
  Bus Selector2/2 -> Virtual Spring/7(xdot2)  "<xdot_AbsEnc>"
  [Kp_s] -> Virtual Spring/2(Kp)
  [Kd_s] -> Virtual Spring/3(Kd)
  Virtual Spring/2(Fs2_1) -> Admittance_BROS2/4(Fext)
  [areConnected] -> Virtual Spring/1(isConnected)
  Admittance_BROS1/4(SPISData) -> [SPISData_BROS1]

== system model_spis/Experiment & Haptics/Subsystem3 ==
  In : Inport
  Enable : EnablePort  StatesWhenEnabling=reset
  Constant : Constant  Value=[0;0]
  Sum2 : Sum  Inputs=++|
  Terminator : Terminator
  pos_boundary : Constant  Value=0.065
  prev_x : UnitDelay  InitialCondition=[0;0]  SampleTime=-1
  vel : Constant  Value=0.15
  virtual mass2 : Constant  Value=FM1.HomeLocationOpSpace
  visuomotor rotation1 : MATLAB Function  TreatAsAtomicUnit=on
  x_ref_square : Outport  InitialOutput=[0;0]
  xdot_ref_square : Outport  Port=2  InitialOutput=[0;0]
  xddot_ref_square : Outport  Port=3  InitialOutput=[0;0]
  wires:
  vel/1 -> visuomotor rotation1/3(vel)
  pos_boundary/1 -> visuomotor rotation1/2(yBound), visuomotor rotation1/1(xBound)
  visuomotor rotation1/1(pos_ref) -> Sum2/2, prev_x/1
  prev_x/1 -> visuomotor rotation1/4(pos_ref_prev)
  visuomotor rotation1/2(vel_ref) -> xdot_ref_square/1
  virtual mass2/1 -> Sum2/1
  Sum2/1 -> x_ref_square/1
  Constant/1 -> xddot_ref_square/1
  In/1 -> Terminator/1

== system model_spis/Experiment & Haptics/Trial Logic ==
  Trial Start Signal : Inport
  Trial Done Signal : Inport  Port=2
  CheckTrialIsRunning : simulink_extras/Flip Flops/S-R Flip-Flop  initial_condition=0
  Data Type Conversion : DataTypeConversion  OutDataTypeStr=double
  Detect Rise Positive : simulink/Logic and Bit Operations/Detect Rise Positive  vinit=0  OutDataTypeStr=boolean
  Detect Rise Positive1 : simulink/Logic and Bit Operations/Detect Rise Positive  vinit=0  OutDataTypeStr=boolean
  Logical Operator : Logic  AllPortsSameDT=off  OutDataTypeStr=boolean
  Memory : Memory
  StopWatch : Subsystem
  Terminator4 : Terminator
  TrialTime : Outport
  TrialRunning : Outport  Port=2
  wires:
  CheckTrialIsRunning/1 -> Memory/1, Data Type Conversion/1
  Memory/1 -> StopWatch/Enable, Logical Operator/1
  Trial Start Signal/1 -> Detect Rise Positive/1
  Detect Rise Positive1/1 -> CheckTrialIsRunning/2
  Detect Rise Positive/1 -> CheckTrialIsRunning/1
  StopWatch/1(trialTime) -> TrialTime/1
  CheckTrialIsRunning/2 -> Terminator4/1
  Data Type Conversion/1 -> TrialRunning/1
  Trial Done Signal/1 -> Logical Operator/2
  Logical Operator/1 -> Detect Rise Positive1/1

== system model_spis/Robot1/AppendToLoggerBus ==
  BusRobot : Inport
  ToEtherCAT_ToLogger : Inport  Port=2
  Controller_ToLogger : Inport  Port=3
  SystemState : Inport  Port=4
  Bus Creator : BusCreator  Inputs=8
  Bus Selector : BusSelector  OutputSignals=xOpSpace,qJointSpace,BusFTSensor,BusActuators
  Bus Selector1 : BusSelector  OutputSignals=ToEtherCAT_ToLogger_Actuator1,ToEtherCAT_ToLogger_Actuator2
  ToLogger : Outport
  wires:
  Bus Creator/1 -> ToLogger/1  "LoggerBus"
  Bus Selector/4 -> Bus Creator/4  "<BusActuators>"
  Bus Selector/1 -> Bus Creator/1  "<xOpSpace>"
  Bus Selector/3 -> Bus Creator/3  "<BusFTSensor>"
  Bus Selector/2 -> Bus Creator/2  "<qJointSpace>"
  BusRobot/1 -> Bus Selector/1
  ToEtherCAT_ToLogger/1 -> Bus Selector1/1
  Bus Selector1/1 -> Bus Creator/5  "<ToEtherCAT_ToLogger_Actuator1>"
  Bus Selector1/2 -> Bus Creator/6  "<ToEtherCAT_ToLogger_Actuator2>"
  Controller_ToLogger/1 -> Bus Creator/7
  SystemState/1 -> Bus Creator/8  "SystemState"

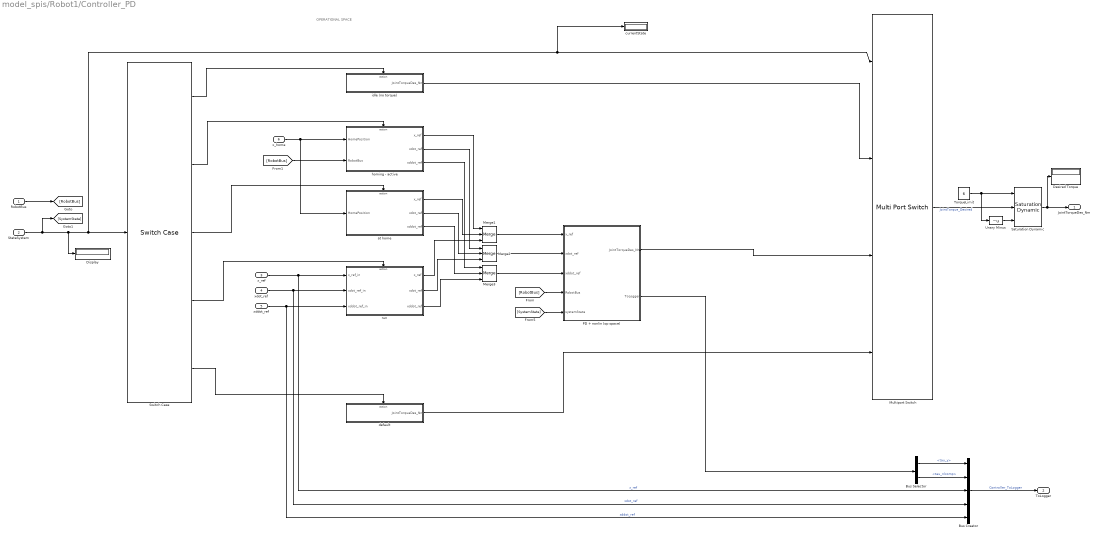
== system model_spis/Robot1/Controller_PD ==
  note: OPERATIONAL SPACE
  RobotBus : Inport
  StateSystem : Inport  Port=2
  x_ref : Inport  Port=3
  xdot_ref : Inport  Port=4
  xddot_ref : Inport  Port=5
  x_home : Inport  Port=6
  Bus Creator : BusCreator  Inputs=5
  Bus Selector : BusSelector  OutputSignals=tau_y,tau_nlcomp
  Desired Torque : Display
  Display : Display
  Merge1 : Merge  Inputs=3  InitialOutput=[0;0]
  Merge2 : Merge  Inputs=3  InitialOutput=[0;0]
  Merge3 : Merge  Inputs=3  InitialOutput=[0;0]
  Multiport Switch : MultiPortSwitch  DataPortOrder=Specify indices  Inputs=4  DataPortIndices={[0,1,2,201,299,301],[302,399,4]}  DataPortForDefault=Additional data port
  PD + nonlin (op space) : Subsystem
  Saturation Dynamic : simulink/Discontinuities/Saturation Dynamic  OutMin=[]  OutMax=[]  OutDataTypeStr=Inherit: Same as second input  OutDataType=fixdt(1, 16)  OutScaling=2^-10  DoSatur=off
  Switch Case : SwitchCase  CaseConditions={[0,1,2,201,299,301],302, 399,[4]}
  TorqueLimit : Constant  Value=6
  Unary Minus : UnaryMinus
  at home : Subsystem
  currentState : Display
  default : Subsystem  TreatAsAtomicUnit=on
  homing - active : Subsystem
  idle (no torque) : Subsystem  TreatAsAtomicUnit=on
  run : Subsystem
  JointTorqueDes_Nm : Outport
  ToLogger : Outport  Port=2
  wires:
  [SystemState] -> PD + nonlin (op space)/5(systemState)
  xddot_ref/1 -> Bus Creator/5, run/3(xddot_ref_in)  "xddot_ref"
  xdot_ref/1 -> Bus Creator/4, run/2(xdot_ref_in)  "xdot_ref"
  x_ref/1 -> Bus Creator/3, run/1(x_ref_in)  "x_ref"
  [RobotBus] -> PD + nonlin (op space)/4(RobotBus)
  RobotBus/1 -> [RobotBus]
  PD + nonlin (op space)/1(JointTorqueDes_Nm) -> Multiport Switch/3
  Merge3/1 -> PD + nonlin (op space)/3(xddot_ref)
  Merge2/1 -> PD + nonlin (op space)/2(xdot_ref)
  Merge1/1 -> PD + nonlin (op space)/1(x_ref)
  idle (no torque)/1(JointTorqueDes_Nm) -> Multiport Switch/2
  Switch Case/2 -> homing - active/Action
  Switch Case/1 -> idle (no torque)/Action
  default/1(JointTorqueDes_Nm) -> Multiport Switch/4
  Switch Case/5 -> default/Action
  Saturation Dynamic/1 -> Desired Torque/1, JointTorqueDes_Nm/1
  Switch Case/3 -> at home/Action
  homing - active/1(x_ref) -> Merge1/1
  run/1(x_ref) -> Merge1/3
  StateSystem/1 -> Display/1, Multiport Switch/1, currentState/1, Switch Case/1, [SystemState]
  run/2(xdot_ref) -> Merge2/3
  run/3(xddot_ref) -> Merge3/3
  homing - active/2(xdot_ref) -> Merge2/1
  homing - active/3(xddot_ref) -> Merge3/1
  Multiport Switch/1 -> Saturation Dynamic/2  "JointTorque_Desired"
  PD + nonlin (op space)/2(ToLogger) -> Bus Selector/1
  x_home/1 -> at home/1(HomePosition), homing - active/1(HomePosition)
  Bus Creator/1 -> ToLogger/1  "Controller_ToLogger"
  Bus Selector/1 -> Bus Creator/1  "<tau_y>"
  Bus Selector/2 -> Bus Creator/2  "<tau_nlcomp>"
  TorqueLimit/1 -> Unary Minus/1, Saturation Dynamic/1
  Unary Minus/1 -> Saturation Dynamic/3
  [RobotBus] -> homing - active/2(RobotBus)
  at home/1(x_ref) -> Merge1/2
  at home/2(xdot_ref) -> Merge2/2
  at home/3(xddot_ref) -> Merge3/2
  Switch Case/4 -> run/Action

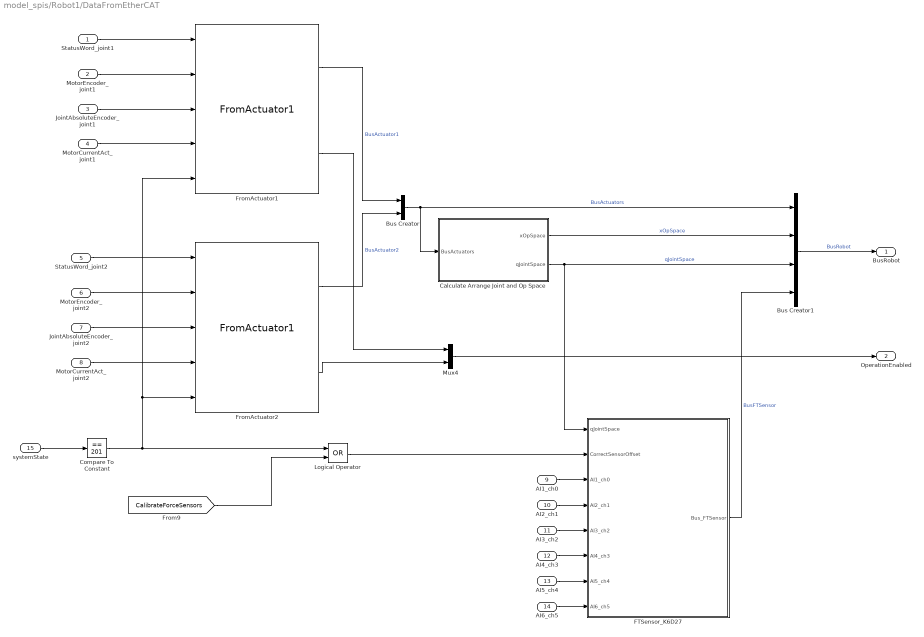
== system model_spis/Robot1/DataFromEtherCAT ==
  StatusWord_joint1 : Inport
  MotorEncoder_joint1 : Inport  Port=2
  JointAbsoluteEncoder_joint1 : Inport  Port=3
  MotorCurrentAct_joint1 : Inport  Port=4
  StatusWord_joint2 : Inport  Port=5
  MotorEncoder_joint2 : Inport  Port=6
  "JointAbsoluteEncoder_joint2 " : Inport  Port=7
  MotorCurrentAct_joint2 : Inport  Port=8
  AI1_ch0 : Inport  Port=9
  AI2_ch1 : Inport  Port=10
  AI3_ch2 : Inport  Port=11
  AI4_ch3 : Inport  Port=12
  AI5_ch4 : Inport  Port=13
  AI6_ch5 : Inport  Port=14
  systemState : Inport  Port=15
  Bus Creator : BusCreator  Inputs=2
  Bus Creator1 : BusCreator  Inputs=4
  Calculate Arrange Joint and Op Space : Subsystem
  Compare To Constant : simulink/Logic and Bit Operations/Compare To Constant  relop===  const=201  OutDataTypeStr=boolean
  FTSensor_K6D27 : Subsystem  mask{FTSensorStruct=RobotStruct.FTSensor}
      mask prompts: FTSensorStruct "Struct for force torque sensor"
  FromActuator1 : LibraryFM/FromActuator1  ActuatorStruct=RobotStruct.Actuator1
  FromActuator2 : LibraryFM/FromActuator1  ActuatorStruct=RobotStruct.Actuator2
  Logical Operator : Logic  Operator=OR  AllPortsSameDT=off  OutDataTypeStr=boolean
  Mux4 : Mux  Inputs=2
  BusRobot : Outport
  OperationEnabled : Outport  Port=2
  wires:
  FTSensor_K6D27/1(Bus_FTSensor) -> Bus Creator1/4  "BusFTSensor"
  FromActuator1/1 -> Bus Creator/1  "BusActuator1"
  FromActuator2/1 -> Bus Creator/2  "BusActuator2"
  FromActuator1/2 -> Mux4/1
  Mux4/1 -> OperationEnabled/1
  FromActuator2/2 -> Mux4/2
  MotorEncoder_joint1/1 -> FromActuator1/2
  StatusWord_joint1/1 -> FromActuator1/1
  JointAbsoluteEncoder_joint1/1 -> FromActuator1/3
  MotorCurrentAct_joint1/1 -> FromActuator1/4
  MotorEncoder_joint2/1 -> FromActuator2/2
  StatusWord_joint2/1 -> FromActuator2/1
  "JointAbsoluteEncoder_joint2 "/1 -> FromActuator2/3
  MotorCurrentAct_joint2/1 -> FromActuator2/4
  Bus Creator/1 -> Calculate Arrange Joint and Op Space/1(BusActuators), Bus Creator1/1  "BusActuators"
  Bus Creator1/1 -> BusRobot/1  "BusRobot"
  Calculate Arrange Joint and Op Space/2(qJointSpace) -> FTSensor_K6D27/1(qJointSpace), Bus Creator1/3  "qJointSpace"
  systemState/1 -> Compare To Constant/1
  AI1_ch0/1 -> FTSensor_K6D27/3(AI1_ch0)
  AI2_ch1/1 -> FTSensor_K6D27/4(AI2_ch1)
  AI3_ch2/1 -> FTSensor_K6D27/5(AI3_ch2)
  AI4_ch3/1 -> FTSensor_K6D27/6(AI4_ch3)
  AI5_ch4/1 -> FTSensor_K6D27/7(AI5_ch4)
  AI6_ch5/1 -> FTSensor_K6D27/8(AI6_ch5)
  Compare To Constant/1 -> FromActuator1/5, FromActuator2/5, Logical Operator/1
  Calculate Arrange Joint and Op Space/1(xOpSpace) -> Bus Creator1/2  "xOpSpace"
  [CalibrateForceSensors] -> Logical Operator/2
  Logical Operator/1 -> FTSensor_K6D27/2(CorrectSensorOffset)

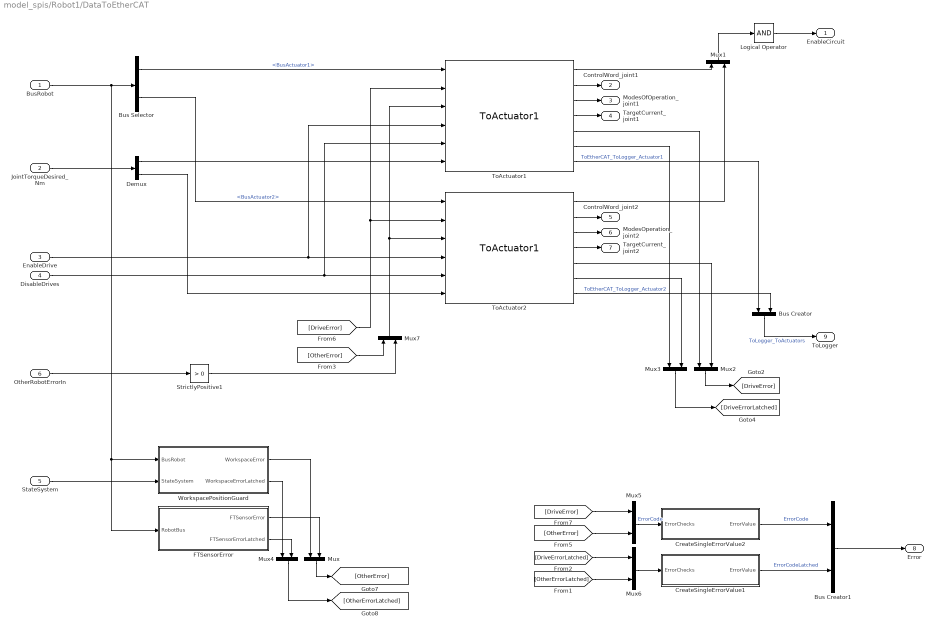
== system model_spis/Robot1/DataToEtherCAT ==
  BusRobot : Inport
  JointTorqueDesired_Nm : Inport  Port=2
  EnableDrive : Inport  Port=3
  DisableDrives : Inport  Port=4
  StateSystem : Inport  Port=5
  OtherRobotErrorIn : Inport  Port=6
  Bus Creator : BusCreator  Inputs=2
  Bus Creator1 : BusCreator  Inputs=2
  Bus Selector : BusSelector  OutputSignals=BusActuators.BusActuator1,BusActuators.BusActuator2
  CreateSingleErrorValue1 : Subsystem
  CreateSingleErrorValue2 : Subsystem
  Demux : Demux  Outputs=2
  FTSensorError : Subsystem
  Logical Operator : Logic  Inputs=1  AllPortsSameDT=off  OutDataTypeStr=boolean
  Mux{,1..7} (8 alike) : Mux  Inputs=2
  StrictlyPositive1 : simulink/Logic and Bit Operations/Compare To Zero  relop=>  OutDataTypeStr=boolean
  ToActuator1 : LibraryFM/ToActuator1  ActuatorStruct=RobotStruct.Actuator1
  ToActuator2 : LibraryFM/ToActuator1  ActuatorStruct=RobotStruct.Actuator2
  WorkspacePositionGuard : Subsystem
  EnableCircuit : Outport  OutDataTypeStr=boolean
  ControlWord_joint1 : Outport  Port=2  OutDataTypeStr=uint16
  ModesOfOperation_joint1 : Outport  Port=3  OutDataTypeStr=int8
  TargetCurrent_joint1 : Outport  Port=4  OutDataTypeStr=int16
  ControlWord_joint2 : Outport  Port=5  OutDataTypeStr=uint16
  ModesOperation_joint2 : Outport  Port=6  OutDataTypeStr=int8
  TargetCurrent_joint2 : Outport  Port=7  OutDataTypeStr=int16
  Error : Outport  Port=8
  ToLogger : Outport  Port=9
  wires:
  Bus Creator/1 -> ToLogger/1  "ToLogger_ToActuators"
  ToActuator2/7 -> Bus Creator/2  "ToEtherCAT_ToLogger_Actuator2"
  ToActuator1/7 -> Bus Creator/1  "ToEtherCAT_ToLogger_Actuator1"
  ToActuator1/5 -> Mux2/1
  ToActuator2/5 -> Mux2/2
  Mux2/1 -> [DriveError]
  ToActuator1/6 -> Mux3/1
  ToActuator2/6 -> Mux3/2
  [DriveError] -> ToActuator1/2, ToActuator2/2
  Mux1/1 -> Logical Operator/1
  ToActuator1/1 -> Mux1/1
  ToActuator2/1 -> Mux1/2
  ToActuator1/2 -> ControlWord_joint1/1
  ToActuator1/3 -> ModesOfOperation_joint1/1
  ToActuator2/2 -> ControlWord_joint2/1
  ToActuator1/4 -> TargetCurrent_joint1/1
  ToActuator2/4 -> TargetCurrent_joint2/1
  ToActuator2/3 -> ModesOperation_joint2/1
  Logical Operator/1 -> EnableCircuit/1
  Demux/2 -> ToActuator2/6
  JointTorqueDesired_Nm/1 -> Demux/1
  Demux/1 -> ToActuator1/6
  BusRobot/1 -> WorkspacePositionGuard/1(BusRobot), FTSensorError/1(RobotBus), Bus Selector/1
  Bus Selector/2 -> ToActuator2/1  "<BusActuator2>"
  Bus Selector/1 -> ToActuator1/1  "<BusActuator1>"
  DisableDrives/1 -> ToActuator1/5, ToActuator2/5
  EnableDrive/1 -> ToActuator1/4, ToActuator2/4
  Mux3/1 -> [DriveErrorLatched]
  StateSystem/1 -> WorkspacePositionGuard/2(StateSystem)
  FTSensorError/1(FTSensorError) -> Mux/2
  FTSensorError/2(FTSensorErrorLatched) -> Mux4/2
  WorkspacePositionGuard/1(WorkspaceError) -> Mux/1
  WorkspacePositionGuard/2(WorkspaceErrorLatched) -> Mux4/1
  Mux/1 -> [OtherError]
  Mux4/1 -> [OtherErrorLatched]
  [DriveError] -> Mux5/1
  [OtherError] -> Mux5/2
  CreateSingleErrorValue1/1(ErrorValue) -> Bus Creator1/2  "ErrorCodeLatched"
  [DriveErrorLatched] -> Mux6/1
  [OtherErrorLatched] -> Mux6/2
  Mux6/1 -> CreateSingleErrorValue1/1(ErrorChecks)
  Mux5/1 -> CreateSingleErrorValue2/1(ErrorChecks)  "ErrorCode"
  Bus Creator1/1 -> Error/1
  CreateSingleErrorValue2/1(ErrorValue) -> Bus Creator1/1  "ErrorCode"
  [OtherError] -> Mux7/1
  Mux7/1 -> ToActuator2/3, ToActuator1/3
  OtherRobotErrorIn/1 -> StrictlyPositive1/1
  StrictlyPositive1/1 -> Mux7/2

== system model_spis/Robot2/AppendToLoggerBus ==
  BusRobot : Inport
  ToEtherCAT_ToLogger : Inport  Port=2
  Controller_ToLogger : Inport  Port=3
  SystemState : Inport  Port=4
  Bus Creator : BusCreator  Inputs=8
  Bus Selector : BusSelector  OutputSignals=xOpSpace,qJointSpace,BusFTSensor,BusActuators
  Bus Selector1 : BusSelector  OutputSignals=ToEtherCAT_ToLogger_Actuator1,ToEtherCAT_ToLogger_Actuator2
  ToLogger : Outport
  wires:
  Bus Creator/1 -> ToLogger/1  "LoggerBus"
  Bus Selector/4 -> Bus Creator/4  "<BusActuators>"
  Bus Selector/1 -> Bus Creator/1  "<xOpSpace>"
  Bus Selector/3 -> Bus Creator/3  "<BusFTSensor>"
  Bus Selector/2 -> Bus Creator/2  "<qJointSpace>"
  BusRobot/1 -> Bus Selector/1
  ToEtherCAT_ToLogger/1 -> Bus Selector1/1
  Bus Selector1/1 -> Bus Creator/5  "<ToEtherCAT_ToLogger_Actuator1>"
  Bus Selector1/2 -> Bus Creator/6  "<ToEtherCAT_ToLogger_Actuator2>"
  Controller_ToLogger/1 -> Bus Creator/7
  SystemState/1 -> Bus Creator/8  "SystemState"

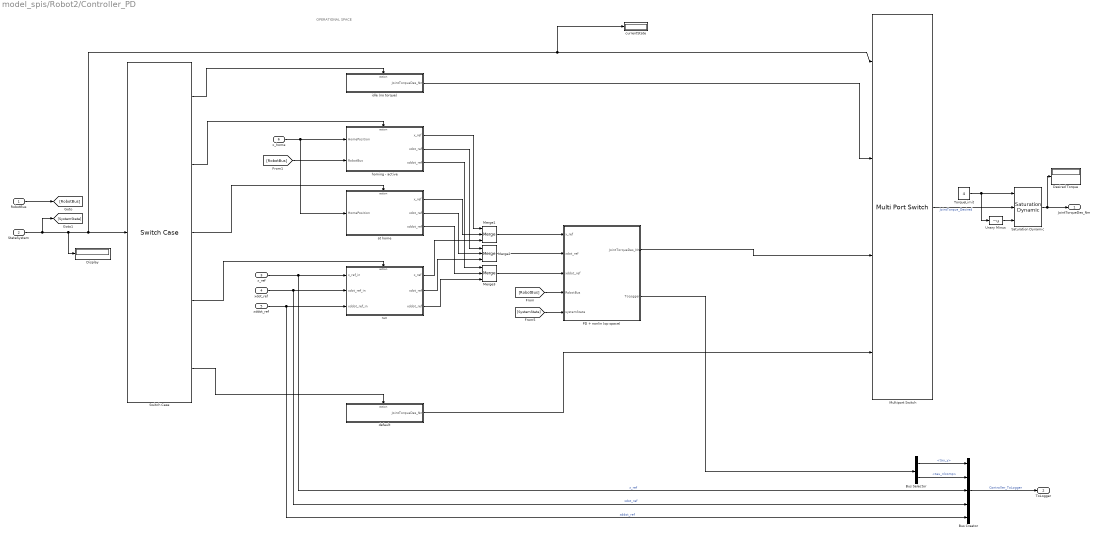
== system model_spis/Robot2/Controller_PD ==
  note: OPERATIONAL SPACE
  RobotBus : Inport
  StateSystem : Inport  Port=2
  x_ref : Inport  Port=3
  xdot_ref : Inport  Port=4
  xddot_ref : Inport  Port=5
  x_home : Inport  Port=6
  Bus Creator : BusCreator  Inputs=5
  Bus Selector : BusSelector  OutputSignals=tau_y,tau_nlcomp
  Desired Torque : Display
  Display : Display
  Merge1 : Merge  Inputs=3  InitialOutput=[0;0]
  Merge2 : Merge  Inputs=3  InitialOutput=[0;0]
  Merge3 : Merge  Inputs=3  InitialOutput=[0;0]
  Multiport Switch : MultiPortSwitch  DataPortOrder=Specify indices  Inputs=4  DataPortIndices={[0,1,2,201,299,301],[302,399,4]}  DataPortForDefault=Additional data port
  PD + nonlin (op space) : Subsystem
  Saturation Dynamic : simulink/Discontinuities/Saturation Dynamic  OutMin=[]  OutMax=[]  OutDataTypeStr=Inherit: Same as second input  OutDataType=fixdt(1, 16)  OutScaling=2^-10  DoSatur=off
  Switch Case : SwitchCase  CaseConditions={[0,1,2,201,299,301],302, 399,[4]}
  TorqueLimit : Constant  Value=4
  Unary Minus : UnaryMinus
  at home : Subsystem
  currentState : Display
  default : Subsystem  TreatAsAtomicUnit=on
  homing - active : Subsystem
  idle (no torque) : Subsystem  TreatAsAtomicUnit=on
  run : Subsystem
  JointTorqueDes_Nm : Outport
  ToLogger : Outport  Port=2
  wires:
  [SystemState] -> PD + nonlin (op space)/5(systemState)
  xddot_ref/1 -> Bus Creator/5, run/3(xddot_ref_in)  "xddot_ref"
  xdot_ref/1 -> Bus Creator/4, run/2(xdot_ref_in)  "xdot_ref"
  x_ref/1 -> Bus Creator/3, run/1(x_ref_in)  "x_ref"
  [RobotBus] -> PD + nonlin (op space)/4(RobotBus)
  RobotBus/1 -> [RobotBus]
  PD + nonlin (op space)/1(JointTorqueDes_Nm) -> Multiport Switch/3
  Merge3/1 -> PD + nonlin (op space)/3(xddot_ref)
  Merge2/1 -> PD + nonlin (op space)/2(xdot_ref)
  Merge1/1 -> PD + nonlin (op space)/1(x_ref)
  idle (no torque)/1(JointTorqueDes_Nm) -> Multiport Switch/2
  Switch Case/2 -> homing - active/Action
  Switch Case/1 -> idle (no torque)/Action
  default/1(JointTorqueDes_Nm) -> Multiport Switch/4
  Switch Case/5 -> default/Action
  Saturation Dynamic/1 -> Desired Torque/1, JointTorqueDes_Nm/1
  Switch Case/3 -> at home/Action
  homing - active/1(x_ref) -> Merge1/1
  run/1(x_ref) -> Merge1/3
  StateSystem/1 -> Display/1, Multiport Switch/1, currentState/1, Switch Case/1, [SystemState]
  run/2(xdot_ref) -> Merge2/3
  run/3(xddot_ref) -> Merge3/3
  homing - active/2(xdot_ref) -> Merge2/1
  homing - active/3(xddot_ref) -> Merge3/1
  Multiport Switch/1 -> Saturation Dynamic/2  "JointTorque_Desired"
  PD + nonlin (op space)/2(ToLogger) -> Bus Selector/1
  x_home/1 -> at home/1(HomePosition), homing - active/1(HomePosition)
  Bus Creator/1 -> ToLogger/1  "Controller_ToLogger"
  Bus Selector/1 -> Bus Creator/1  "<tau_y>"
  Bus Selector/2 -> Bus Creator/2  "<tau_nlcomp>"
  TorqueLimit/1 -> Unary Minus/1, Saturation Dynamic/1
  Unary Minus/1 -> Saturation Dynamic/3
  [RobotBus] -> homing - active/2(RobotBus)
  at home/1(x_ref) -> Merge1/2
  at home/2(xdot_ref) -> Merge2/2
  at home/3(xddot_ref) -> Merge3/2
  Switch Case/4 -> run/Action
